simulink model "ask"  (R2018b)
settings: Solver=VariableStepAuto  StartTime=0.0  StopTime=10.0  MaxStep=0.001  RelTol=1e-3
libraries: simulink x1
settings Model: Creator=sin  LastModifiedBy=sin

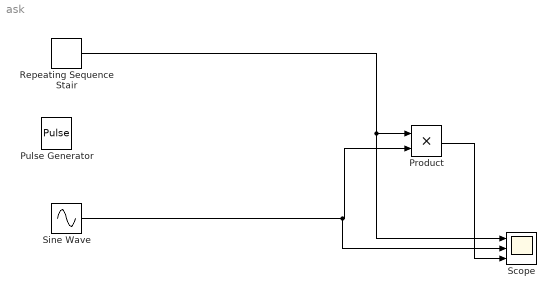
== system ask ==
  Product : Product
  Pulse Generator : DiscretePulseGenerator  PulseType=Time based  PulseWidth=50
  Repeating Sequence Stair : simulink/Sources/Repeating Sequence Stair  OutValues=[0 0 1 1 0 1 1 0 0 1].'  tsamp=1  OutMin=[]  OutMax=[]  OutDataTypeStr=double  OutputDataTypeScalingMode=double  OutDataType=fixdt(0,8)  ConRadixGroup=Best Precision: Vector-wise  OutScaling=2^-12
  Scope : Scope  NumInputPorts=3
  Sine Wave : Sin  Frequency=2*2*pi  SampleTime=0
  wires:
  Repeating Sequence Stair/1 -> Scope/1, Product/1
  Product/1 -> Scope/3
  Sine Wave/1 -> Scope/2, Product/2
